simulink model "fft_2pt_co_sim"  (Simulink 8.0)
settings: Solver=FixedStepDiscrete  SolverMode=SingleTasking  StartTime=0.0  StopTime=50  RelTol=1e-3
libraries: xbsIndex_r4 x13
settings Model: Creator=dell  LastModifiedBy=dell

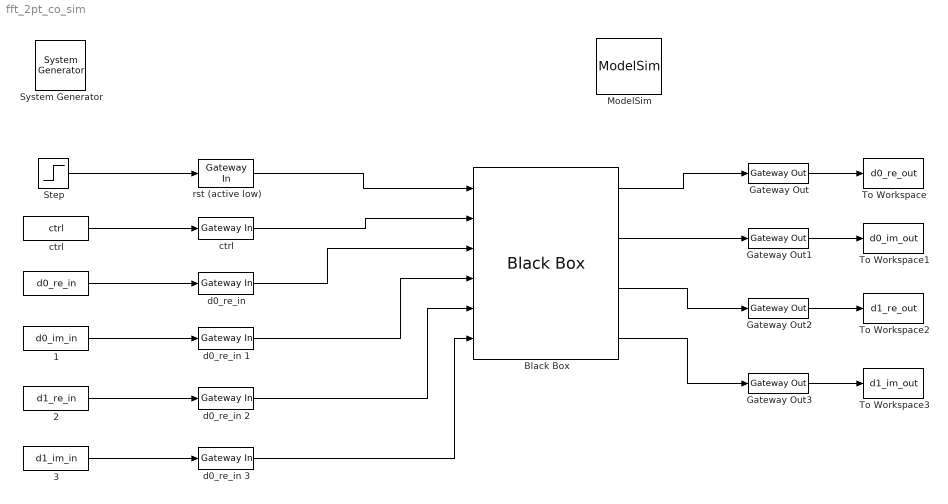
== system fft_2pt_co_sim ==
  " " : FromWorkspace  VariableName=d0_re_in  SampleTime=1
  " 1" : FromWorkspace  VariableName=d0_im_in  SampleTime=1
  " 2" : FromWorkspace  VariableName=d1_re_in  SampleTime=1
  " 3" : FromWorkspace  VariableName=d1_im_in  SampleTime=1
  " System Generator" : xbsIndex_r4/ System Generator  Tag=genX  xilinxfamily=Kintex7  part=xc7k325t  speed=-3  package=fbg676  synthesis_tool=XST  clock_wrapper=Clock Enables  directory=./netlist  proj_type=Project Navigator  Synth_file=XST Defaults  Impl_file=ISE Defaults  testbench=off  simulink_period=1  sysclk_period=10  dcm_input_clock_period=10  incr_netlist=off  trim_vbits=Everywhere in SubSystem  dbl_ovrd=According to Block Masks  core_generation=According to Block Masks  run_coregen=off  deprecated_control=off  eval_field=0  block_type=sysgen
  Black Box : xbsIndex_r4/Black Box  init_code=fft_pt2_config  sim_method=External co-simulator  engine_block=ModelSim  verbose=off  block_type=blackbox2
  Gateway Out{,1..3} (4 alike) : xbsIndex_r4/Gateway Out  inherit_from_input=off  hdl_port=on  timing_constraint=None  locs_specified=off  LOCs={}  UseAsDAC=off  DACChannel='1'  block_type=gatewayout
  ModelSim : xbsIndex_r4/ModelSim  dir=./modelsim  waveform=on  leave_open=on  skip_compile=off  use_unisim=off  use_ver_xilinxcorelib=off  custom_scripts=on  vsim_script=vsim_instead.do  post_vsim_script=./before.do  startup_timeout=40  block_type=hdlcosim
      settings: infoedit="Allow other blocks to schedule HDL co-simulation tasks.<br><br>Note that selecting \"Skip compilation\" when inappropriate can cause simulation errors and failures. Please refer to the block help for details."
  Step : Step  SampleTime=1
  To Workspace : ToWorkspace  VariableName=d0_re_out  SampleTime=-1  SaveFormat=Timeseries
  To Workspace1 : ToWorkspace  VariableName=d0_im_out  SampleTime=-1  SaveFormat=Timeseries
  To Workspace2 : ToWorkspace  VariableName=d1_re_out  SampleTime=-1  SaveFormat=Timeseries
  To Workspace3 : ToWorkspace  VariableName=d1_im_out  SampleTime=-1  SaveFormat=Timeseries
  ctrl : FromWorkspace  VariableName=ctrl  SampleTime=1
  "ctrl " : xbsIndex_r4/Gateway In  gui_display_data_type=Boolean  arith_type=Boolean  n_bits=16  bin_pt=0  preci_type=Single  exp_width=8  frac_width=24  quantization="Round  (unbiased: +/- Inf)"  overflow=Saturate  period=1  dbl_ovrd=off  timing_constraint=None  locs_specified=off  LOCs={}  UseAsADC=off  ADCChannel='1'  inherit_from_input=off  hdl_port=on  block_type=gatewayin
      settings: xl_area=[0, 0, 0, 0, 0, 0, 0]  block_version=VER_STRING_GOES_HERE
  d0_re_in {,1..3} (4 alike) : xbsIndex_r4/Gateway In  gui_display_data_type=Boolean  arith_type=Boolean  n_bits=10  bin_pt=8  preci_type=Single  exp_width=8  frac_width=24  quantization="Round  (unbiased: +/- Inf)"  overflow=Saturate  period=1  dbl_ovrd=off  timing_constraint=None  locs_specified=off  LOCs={}  UseAsADC=off  ADCChannel='1'  inherit_from_input=off  hdl_port=on  block_type=gatewayin
      settings: xl_area=[0, 0, 0, 0, 0, 0, 0]  block_version=VER_STRING_GOES_HERE
  rst (active low) : xbsIndex_r4/Gateway In  gui_display_data_type=Boolean  arith_type=Boolean  n_bits=10  bin_pt=8  preci_type=Single  exp_width=8  frac_width=24  quantization="Round  (unbiased: +/- Inf)"  overflow=Saturate  period=1  dbl_ovrd=off  timing_constraint=None  locs_specified=off  LOCs={}  UseAsADC=off  ADCChannel='1'  inherit_from_input=off  hdl_port=on  block_type=gatewayin
      settings: xl_area=[0, 0, 0, 0, 0, 0, 0]  block_version=VER_STRING_GOES_HERE
  wires:
  Step/1 -> rst (active low)/1
  ctrl/1 -> "ctrl "/1
  " "/1 -> "d0_re_in "/1
  "ctrl "/1 -> Black Box/2
  "d0_re_in "/1 -> Black Box/3
  rst (active low)/1 -> Black Box/1
  " 1"/1 -> d0_re_in 1/1
  d0_re_in 1/1 -> Black Box/4
  " 2"/1 -> d0_re_in 2/1
  d0_re_in 2/1 -> Black Box/5
  " 3"/1 -> d0_re_in 3/1
  d0_re_in 3/1 -> Black Box/6
  Black Box/1 -> Gateway Out/1
  Black Box/2 -> Gateway Out1/1
  Black Box/3 -> Gateway Out2/1
  Black Box/4 -> Gateway Out3/1
  Gateway Out/1 -> To Workspace/1
  Gateway Out1/1 -> To Workspace1/1
  Gateway Out2/1 -> To Workspace2/1
  Gateway Out3/1 -> To Workspace3/1
